simulink model "Filtering_PI_PreliminarySimulation"  (R2025a)
settings: Solver=VariableStepAuto  StartTime=0.0  StopTime=0.5  MaxStep=1e-4  RelTol=1e-3
undefined symbols (not defined in the file): D1, lagging, pulse
libraries: spsSeriesRLCBranchLib x43, spsGroundLib x17, spsMeanLib x1, spsMultimeterLib x1, slpidlib x1, spsPLL3phLib x1, spsPower3phInstantaneousLib x1, spsPulseGeneratorThyristor6PulseLib x1, spsRMSLib x1, simulink x1, spsThreePhaseProgrammableVoltageSourceLib x1, spsThreePhaseSeriesRLCBranchLib x1
settings Model: Creator=wz  LastModifiedBy=wz

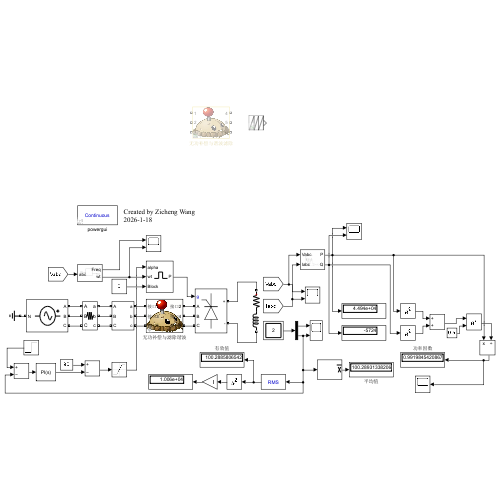
[thumbnail: Simulink's stored preview of the top-level diagram]
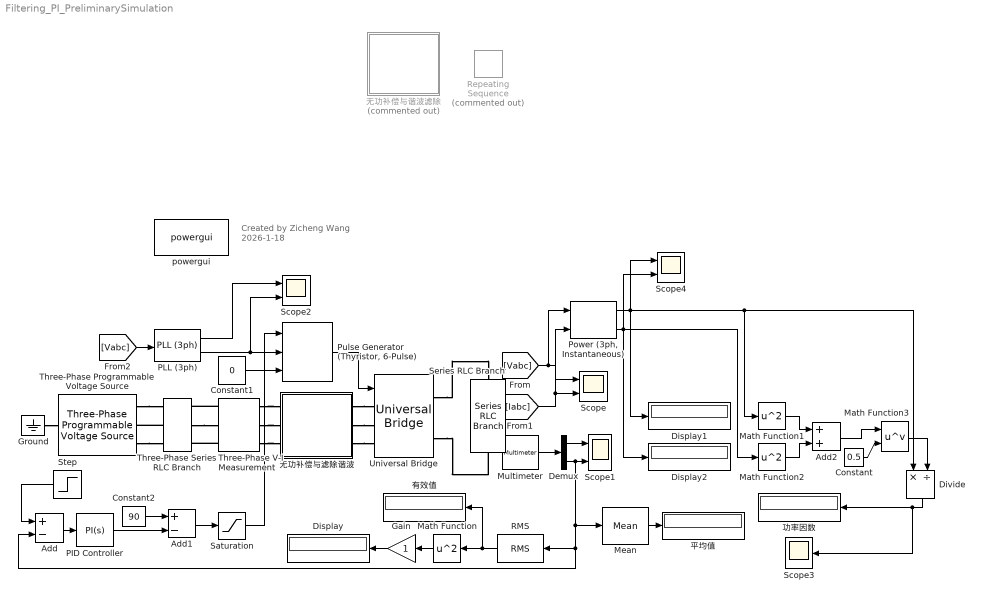
== system Filtering_PI_PreliminarySimulation ==
  note: Created by Zicheng Wang
      | 2026-1-18
  Add : Sum  Inputs=+-
  Add1 : Sum  Inputs=+-
  Add2 : Sum
  Constant : Constant  Value=0.5
  Constant1 : Constant  Value=0
  Constant2 : Constant  Value=90
  Demux : Demux  Outputs=2
  Display : Display
  Display1 : Display
  Display2 : Display
  Divide : Product  Inputs=*/
  Gain : Gain
  Ground : spsGroundLib/Ground  LConnTagsString=a
  Math Function : Math  Operator=square
  Math Function1 : Math  Operator=square
  Math Function2 : Math  Operator=square
  Math Function3 : Math  Operator=pow
  Mean : spsMeanLib/Mean  Freq=60  Vinit=0  Ts=0
  Multimeter : spsMultimeterLib/Multimeter  L=2  sel=[1 2]  yselected={}  Gain=[1 1]  OutputType=Complex  PlotAtSimulationStop=off  PhasorSimulation=off
  PID Controller : slpidlib/PID Controller  Controller=PI  Form=Parallel  TimeDomain=Continuous-time  UseExternalTs=off  SampleTime=-1  IntegratorMethod=Forward Euler  FilterMethod=Forward Euler  ControllerParametersSource=internal  P=2  I=0.5  UseKiTs=off  D=0  UseExternalDerivativeSource=off  N=100  UseFilter=on  TunerSelectOption=Transfer Function Based (PID Tuner App)  InitialConditionSource=internal  InitialConditionForIntegrator=0  InitialConditionForFilter=0  DifferentiatorICPrevScaledInput=0  ExternalReset=none  TrackingMode=off  Kt=1  LimitOutput=off  SatLimitsSource=internal  UpperSaturationLimit=inf  LowerSaturationLimit=-inf  LinearizeAsGain=on  AntiWindupMode=none  Kb=1  LimitIntegrator=off  UpperIntegratorSaturationLimit=inf  LowerIntegratorSaturationLimit=-inf  POutMin=[]  POutMax=[]  IOutMin=[]  IOutMax=[]  DOutMin=[]  DOutMax=[]  NOutMin=[]  NOutMax=[]  SumOutMin=[]  SumOutMax=[]  SaturationOutMin=[]  SaturationOutMax=[]  PParamMin=[]  PParamMax=[]  IParamMin=[]  IParamMax=[]  DParamMin=[]  DParamMax=[]  NParamMin=[]  NParamMax=[]  KbParamMin=[]  KbParamMax=[]  KtParamMin=[]  KtParamMax=[]  KbOutMin=[]  KbOutMax=[]  KtOutMin=[]  KtOutMax=[]  IntegratorOutMin=[]  IntegratorOutMax=[]  FilterOutMin=[]  FilterOutMax=[]  SumI1OutMin=[]  SumI1OutMax=[]  SumI2OutMin=[]  SumI2OutMax=[]  SumI3OutMin=[]  SumI3OutMax=[]  SumI4OutMin=[]  SumI4OutMax=[]  SumDOutMin=[]  SumDOutMax=[]  DifferentiatorOutMin=[]  DifferentiatorOutMax=[]  FilterDiffOutCoefMin=[]  FilterDiffOutCoefMax=[]  ReciprocalOutMin=[]  ReciprocalOutMax=[]  SumDenOutMin=[]  SumDenOutMax=[]  SumNumOutMin=[]  SumNumOutMax=[]  DivideOutMin=[]  DivideOutMax=[]  UdiffTsProdOutMin=[]  UdiffTsProdOutMax=[]  NTsProdOutMin=[]  NTsProdOutMax=[]  UintegralTsProdOutMin=[]  UintegralTsProdOutMax=[]  UngainTsProdOutMin=[]  UngainTsProdOutMax=[]  ClampingZeroOutDataTypeStr=Inherit: Inherit via back propagation  ClampingZeroOutMin=[]  ClampingZeroOutMax=[]  FilterDenConstantOutDataTypeStr=Inherit: Inherit via back propagation  FilterDenConstantOutMin=[]  FilterDenConstantOutMax=[]  PCopyOutDataTypeStr=Inherit: Inherit via back propagation  PCopyOutMin=[]  PCopyOutMax=[]  NCopyOutDataTypeStr=Inherit: Inherit via back propagation  NCopyOutMin=[]  NCopyOutMax=[]  IntegratorContinuousStateAttributes=''  IntegratorStateMustResolveToSignalObject=off  IntegratorRTWStateStorageClass=Auto  FilterContinuousStateAttributes=''  FilterStateMustResolveToSignalObject=off  FilterRTWStateStorageClass=Auto  ParallelPVariant=InternalParameters  IdealPVariant=Disabled  IVariant=InternalParameters  DVariant=Disabled  IntegratorVariant=Continuous  SatVariant=Disabled  AWVariant=Passthrough  PCopyVariant=Disabled  TRVariant=Disabled  FdbkBlocksVariant=Forward  IdealPFdbkVariant=Disabled  SatFdbkVariant=Disabled  DerivativeFilterVariant=Disabled  NVariant=Disabled  NCopyVariant=Disabled_SignalSpec  FilterICVariant=Disabled  IntegratorICVariant=InternalICs  ExternalResetVariant=Disabled  TRSumVariant=Passthrough  SumFdbkVariant=Disabled  SumVariant=Sum_PI  TsampFilterVariant=InternalTs  TsampNgainVariant=Passthrough  TsampIntegralVariant=Disabled_SignalSpec  ExternalSaturationOutDataTypeStr=Inherit: Same as second input  DerivativeSourceVariant=Disabled  PreIntVariant=InternalPreInt
  PLL (3ph) : spsPLL3phLib/PLL (3ph)  Fmin=49  Par_Init=[0, 50]  ParK=[180, 3200, 1]  TcD=1e-4  MaxRateChangeFreq=12  FilterCutOffFreq=25  Ts=0  AGC=on
  "Power (3ph, Instantaneous)" : spsPower3phInstantaneousLib/Power (3ph, Instantaneous)
  "Pulse Generator (Thyristor, 6-Pulse)" : spsPulseGeneratorThyristor6PulseLib/Pulse Generator (Thyristor, 6-Pulse)  GenType=6-pulse  Delta=D1 (lagging)  pwidth=60  Double_Pulse=off  Ts=0
      settings: LibrarySourceBlock=|
      | sps_lib/Power Electronics/Power Electronics Control/Pulse Generator
      | (Thyristor, 6-Pulse)
  RMS : spsRMSLib/RMS  TrueRMS=on  Freq=50  RMSInit=120  Ts=0
  Repeating Sequence : simulink/Sources/Repeating Sequence  Commented=on  rep_seq_t=[0 1/50]  rep_seq_y=[0 2*pi]
  Saturation : Saturate  UpperLimit=90  LowerLimit=0
  Scope{,1..2,4} (4 alike) : Scope  NumInputPorts=2
      Scope settings: ActiveDisplayYMinimum=-1  ActiveDisplayYMaximum=1
      Scope1 settings: ActiveDisplayYMinimum=-51.707918022923707  ActiveDisplayYMaximum=59.934540956922731
      Scope2 settings: ActiveDisplayYMinimum=-1  ActiveDisplayYMaximum=1  DataLoggingVariableName=ScopeData2
      Scope4 settings: ActiveDisplayYMinimum=-1  ActiveDisplayYMaximum=1  DataLoggingVariableName=ScopeData4
  Scope3 : Scope
      settings: ActiveDisplayYMinimum=0.98403716767059757  ActiveDisplayYMaximum=0.9967412923994573  DataLoggingVariableName=ScopeData3
  Series RLC Branch : spsSeriesRLCBranchLib/Series RLC Branch  LConnTagsString=__new0  RConnTagsString=__new0  BranchType=RL  Resistance=0.01  Inductance=0.025  SetiL0=off  InitialCurrent=0  Capacitance=1e-6  Setx0=off  InitialVoltage=0  Measurements=Branch voltage and current
  Step : Step  Time=0.02  After=105  SampleTime=0
  Three-Phase Programmable Voltage Source : spsThreePhaseProgrammableVoltageSourceLib/Three-Phase Programmable Voltage Source  PositiveSequence="[380  0 50]"  VariationEntity=None  VariationType=Table of time-amplitude pairs  VariationTypeAlt=Step  VariationStep=0.5  VariationRate=10  VariationMagnitude=0.3  VariationFrequency=2  VariationTiming=[1 2]  VariationPhaseA=off  Amplitudes=[1 0.8 1.2 1.0]  TimeValues=[0 0.1 0.15 0.2]  HarmonicGeneration=off  HarmonicA=[3 0.2 -25 0]  HarmonicB=[2 0.15 35 2]  Timing="[0.05  3]"  BusType=swing  Pref=0  Qref=0  Qmin=-inf  Qmax=inf
  Three-Phase Series RLC Branch : spsThreePhaseSeriesRLCBranchLib/Three-Phase Series RLC Branch  LConnTagsString=A|B|C  RConnTagsString=A|B|C  BranchType=R  Resistance=0.01  Inductance=1e-3  Capacitance=1e-6  Measurements=None
  Three-Phase V-I Measurement : spsThreePhaseVIMeasurementLib/Three-Phase V-I Measurement  VoltageMeasurement=phase-to-ground  SetLabelV=on  LabelV=Vabc  Vpu=off  VpuLL=off  CurrentMeasurement=yes  SetLabelI=on  LabelI=Iabc  Ipu=off  Pbase=100e6  Vbase=500e3  OutputType=Complex  PhasorSimulation=off  PSBequivalent=0
  Universal Bridge : spsUniversalBridgeLib/Universal Bridge  Arms=3  SnubberResistance=1e5  SnubberCapacitance=inf  Device=Thyristors  Ron=1e-3  Lon=0  ForwardVoltages="[  0  0  ]"  ForwardVoltage=0  GTOparameters=[ 10e-6 , 20e-6 ]  IGBTparameters=[ 1e-6 , 2e-6 ]  Measurements=None  Measurements_2=None  converterType=Rectifier
  powergui : sps_lib/powergui  Priority=1  SimulationMode=Continuous  SampleTime=50e-6  frequency=60  Iterations=50  frequencyindice=50  Pbase=100e6  ErrMax=1e-4  UnitsV=kV  UnitsW=MW  buscounter=0  FunctionMessages=off  echomessages=off  EnableUseOfTLC=off  CurrentSourceSwitches=off  DisableSnubberDevices=off  DisableRonSwitches=off  DisableVfSwitches=off  DisplayEquations=off  AutomaticDiscreteSolvers=off  SolverType=Tustin/Backward Euler (TBE)  Interpol=off  ExternalGateDelay=off  methode=off  Ts=100  x0status=blocks  SPID=on  SwTol=0  HookPort=off  NonlinearTolerance=1e-4  nMaxIteration=100  ContinueOnMaxIteration=off  RestoreLinks=warning  ResistiveCurrentMeasurement=off  Frange=[0:2:500]  Ylog=off  Xlog=on  ShowGrid=off  save=off  variable=ZData  structure=0  ZoomFFT=off  StartTime=0.0  cycles=1  DisplayStyle=1  fundamental=60  FreqAxis=off  MaxFrequency=1000  frequencyindicesteady=1  RmsSteady=1  display=off
  功率因数 : Display
  平均值 : Display
  无功补偿与滤除谐波 : Subsystem  mask{R0=1.2, R1=0.65, R2=0.65, R3=0.45, CLBQ1=1e-2, RLBQ1=0.0001, LLBQ1=4.05284734569351, CLBQ2=3e-4, RLBQ2=1e-6, LLBQ2=0.000689259752668965, CLBQ3=3e-3, RLBQ3=1e-4, LLBQ3=0.000279121718022969, CLBQ4=5e-3, RLBQ4=0.3, LLBQ4=0.0059953363101975/5, CLBQ5=10, RLBQ5=50, LLBQ5=3.50592330942345}
      mask prompts: R0 "R0value1"; R1 "R0value2"; R2 "R0value3"; R3 "R0value4"; CLBQ1 "CLBQvalue1"; RLBQ1 "RLBQvalue1"; LLBQ1 "LLBQvalue1"; CLBQ2 "CLBQvalue2"; RLBQ2 "RLBQvalue2"; LLBQ2 "LLBQvalue2"; CLBQ3 "CLBQvalue3"; RLBQ3 "RLBQvalue3"; LLBQ3 "LLBQvalue3"; CLBQ4 "CLBQvalue4"; RLBQ4 "RLBQvalue4"; LLBQ4 "LLBQvalue4"; CLBQ5 "CLBQvalue5"; RLBQ5 "RLBQvalue5"; LLBQ5 "LLBQvalue5"
      mask Display: image('微信图片_20240530165846.jpg');
  无功补偿与谐波滤除 : Subsystem  Commented=on
      mask DialogControl DescTextVar Prompt: 单调
      mask DialogControl ParameterGroupVar Prompt: 参数
      mask Display: image('微信图片_20240530165846.jpg');
  有效值 : Display
  wires:
  Constant1/1 -> "Pulse Generator (Thyristor, 6-Pulse)"/3
  [Vabc] -> "Power (3ph, Instantaneous)"/1, Scope/1
  [Iabc] -> "Power (3ph, Instantaneous)"/2, Scope/2
  PLL (3ph)/2 -> Scope2/2, "Pulse Generator (Thyristor, 6-Pulse)"/2
  "Pulse Generator (Thyristor, 6-Pulse)"/1 -> Universal Bridge/1
  [Vabc] -> PLL (3ph)/1
  PLL (3ph)/1 -> Scope2/1
  Multimeter/1 -> Demux/1
  Demux/1 -> Scope1/1
  Demux/2 -> Mean/1, Add/2, RMS/1, Scope1/2
  Add/1 -> PID Controller/1
  PID Controller/1 -> Add1/2
  Constant2/1 -> Add1/1
  Add1/1 -> Saturation/1
  Saturation/1 -> "Pulse Generator (Thyristor, 6-Pulse)"/1
  RMS/1 -> 有效值/1, Math Function/1
  Math Function/1 -> Gain/1
  Gain/1 -> Display/1
  "Power (3ph, Instantaneous)"/1 -> Scope4/1, Divide/1, Math Function1/1, Display1/1
  "Power (3ph, Instantaneous)"/2 -> Scope4/2, Math Function2/1, Display2/1
  Step/1 -> Add/1
  Math Function1/1 -> Add2/1
  Math Function2/1 -> Add2/2
  Add2/1 -> Math Function3/1
  Constant/1 -> Math Function3/2
  Math Function3/1 -> Divide/2
  Divide/1 -> Scope3/1, 功率因数/1
  Mean/1 -> 平均值/1
  connections:
  Universal Bridge/RConn1 -- Series RLC Branch/LConn1
  Universal Bridge/RConn2 -- Series RLC Branch/RConn1
  Ground/LConn1 -- Three-Phase Programmable Voltage Source/LConn1
  无功补偿与滤除谐波/RConn1 -- Universal Bridge/LConn1
  无功补偿与滤除谐波/RConn2 -- Universal Bridge/LConn2
  无功补偿与滤除谐波/RConn3 -- Universal Bridge/LConn3
  Three-Phase V-I Measurement/RConn1 -- 无功补偿与滤除谐波/LConn1
  Three-Phase V-I Measurement/RConn2 -- 无功补偿与滤除谐波/LConn2
  Three-Phase V-I Measurement/RConn3 -- 无功补偿与滤除谐波/LConn3
  Three-Phase Programmable Voltage Source/RConn1 -- Three-Phase Series RLC Branch/LConn1
  Three-Phase V-I Measurement/LConn1 -- Three-Phase Series RLC Branch/RConn1
  Three-Phase Series RLC Branch/LConn2 -- Three-Phase Programmable Voltage Source/RConn2
  Three-Phase Programmable Voltage Source/RConn3 -- Three-Phase Series RLC Branch/LConn3
  Three-Phase Series RLC Branch/RConn2 -- Three-Phase V-I Measurement/LConn2
  Three-Phase V-I Measurement/LConn3 -- Three-Phase Series RLC Branch/RConn3

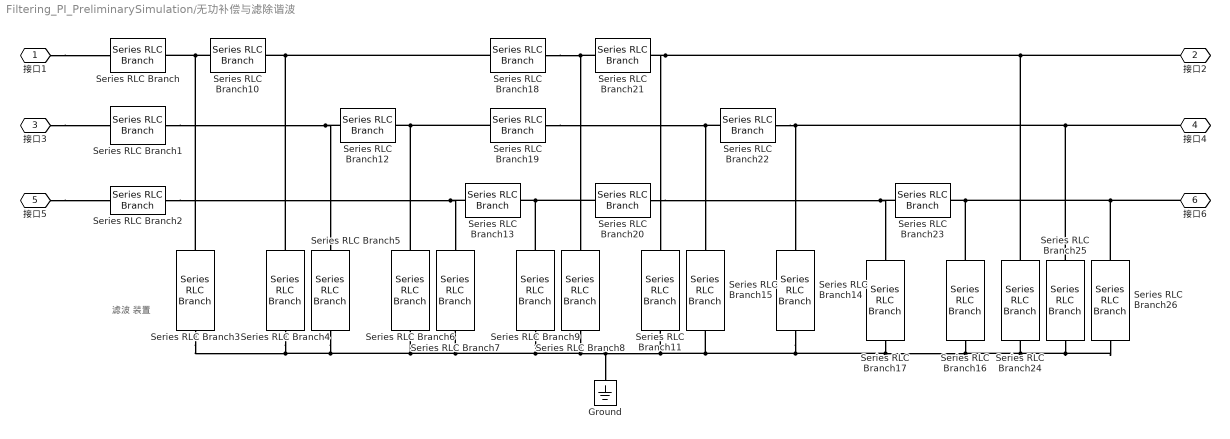
== system Filtering_PI_PreliminarySimulation/无功补偿与滤除谐波 ==
  note: 滤波
      | 装置
  Ground : spsGroundLib/Ground  LConnTagsString=a
  Series RLC Branch : spsSeriesRLCBranchLib/Series RLC Branch  LConnTagsString=__new0  RConnTagsString=__new0  BranchType=R  Resistance=R0  Inductance=1e-3  SetiL0=off  InitialCurrent=0  Capacitance=1e-6  Setx0=off  InitialVoltage=0  Measurements=None
  Series RLC Branch1 : spsSeriesRLCBranchLib/Series RLC Branch  LConnTagsString=__new0  RConnTagsString=__new0  BranchType=R  Resistance=R0  Inductance=1e-3  SetiL0=off  InitialCurrent=0  Capacitance=1e-6  Setx0=off  InitialVoltage=0  Measurements=None
  Series RLC Branch10 : spsSeriesRLCBranchLib/Series RLC Branch  LConnTagsString=__new0  RConnTagsString=__new0  BranchType=R  Resistance=R1  Inductance=1e-3  SetiL0=off  InitialCurrent=0  Capacitance=1e-6  Setx0=off  InitialVoltage=0  Measurements=None
  Series RLC Branch11 : spsSeriesRLCBranchLib/Series RLC Branch  LConnTagsString=__new0  RConnTagsString=__new0  BranchType=RLC  Resistance=RLBQ4  Inductance=LLBQ4  SetiL0=off  InitialCurrent=0  Capacitance=CLBQ4  Setx0=off  InitialVoltage=0  Measurements=None
  Series RLC Branch12 : spsSeriesRLCBranchLib/Series RLC Branch  LConnTagsString=__new0  RConnTagsString=__new0  BranchType=R  Resistance=R1  Inductance=1e-3  SetiL0=off  InitialCurrent=0  Capacitance=1e-6  Setx0=off  InitialVoltage=0  Measurements=None
  Series RLC Branch13 : spsSeriesRLCBranchLib/Series RLC Branch  LConnTagsString=__new0  RConnTagsString=__new0  BranchType=R  Resistance=R1  Inductance=1e-3  SetiL0=off  InitialCurrent=0  Capacitance=1e-6  Setx0=off  InitialVoltage=0  Measurements=None
  Series RLC Branch14 : spsSeriesRLCBranchLib/Series RLC Branch  LConnTagsString=__new0  RConnTagsString=__new0  BranchType=RLC  Resistance=RLBQ4  Inductance=LLBQ4  SetiL0=off  InitialCurrent=0  Capacitance=CLBQ4  Setx0=off  InitialVoltage=0  Measurements=None
  Series RLC Branch15 : spsSeriesRLCBranchLib/Series RLC Branch  LConnTagsString=__new0  RConnTagsString=__new0  BranchType=RLC  Resistance=RLBQ3  Inductance=LLBQ3  SetiL0=off  InitialCurrent=0  Capacitance=CLBQ3  Setx0=off  InitialVoltage=0  Measurements=None
  Series RLC Branch16 : spsSeriesRLCBranchLib/Series RLC Branch  LConnTagsString=__new0  RConnTagsString=__new0  BranchType=RLC  Resistance=RLBQ4  Inductance=LLBQ4  SetiL0=off  InitialCurrent=0  Capacitance=CLBQ4  Setx0=off  InitialVoltage=0  Measurements=None
  Series RLC Branch17 : spsSeriesRLCBranchLib/Series RLC Branch  LConnTagsString=__new0  RConnTagsString=__new0  BranchType=RLC  Resistance=RLBQ3  Inductance=LLBQ3  SetiL0=off  InitialCurrent=0  Capacitance=CLBQ3  Setx0=off  InitialVoltage=0  Measurements=None
  Series RLC Branch18 : spsSeriesRLCBranchLib/Series RLC Branch  LConnTagsString=__new0  RConnTagsString=__new0  BranchType=R  Resistance=R2  Inductance=1e-3  SetiL0=off  InitialCurrent=0  Capacitance=1e-6  Setx0=off  InitialVoltage=0  Measurements=None
  Series RLC Branch19 : spsSeriesRLCBranchLib/Series RLC Branch  LConnTagsString=__new0  RConnTagsString=__new0  BranchType=R  Resistance=R2  Inductance=1e-3  SetiL0=off  InitialCurrent=0  Capacitance=1e-6  Setx0=off  InitialVoltage=0  Measurements=None
  Series RLC Branch2 : spsSeriesRLCBranchLib/Series RLC Branch  LConnTagsString=__new0  RConnTagsString=__new0  BranchType=R  Resistance=R0  Inductance=1e-3  SetiL0=off  InitialCurrent=0  Capacitance=1e-6  Setx0=off  InitialVoltage=0  Measurements=None
  Series RLC Branch20 : spsSeriesRLCBranchLib/Series RLC Branch  LConnTagsString=__new0  RConnTagsString=__new0  BranchType=R  Resistance=R2  Inductance=1e-3  SetiL0=off  InitialCurrent=0  Capacitance=1e-6  Setx0=off  InitialVoltage=0  Measurements=None
  Series RLC Branch21 : spsSeriesRLCBranchLib/Series RLC Branch  LConnTagsString=__new0  RConnTagsString=__new0  BranchType=R  Resistance=R3  Inductance=1e-3  SetiL0=off  InitialCurrent=0  Capacitance=1e-6  Setx0=off  InitialVoltage=0  Measurements=None
  Series RLC Branch22 : spsSeriesRLCBranchLib/Series RLC Branch  LConnTagsString=__new0  RConnTagsString=__new0  BranchType=R  Resistance=R3  Inductance=1e-3  SetiL0=off  InitialCurrent=0  Capacitance=1e-6  Setx0=off  InitialVoltage=0  Measurements=None
  Series RLC Branch23 : spsSeriesRLCBranchLib/Series RLC Branch  LConnTagsString=__new0  RConnTagsString=__new0  BranchType=R  Resistance=R3  Inductance=1e-3  SetiL0=off  InitialCurrent=0  Capacitance=1e-6  Setx0=off  InitialVoltage=0  Measurements=None
  Series RLC Branch24 : spsSeriesRLCBranchLib/Series RLC Branch  LConnTagsString=__new0  RConnTagsString=__new0  BranchType=RLC  Resistance=RLBQ5  Inductance=LLBQ5  SetiL0=off  InitialCurrent=0  Capacitance=CLBQ5  Setx0=off  InitialVoltage=0  Measurements=None
  Series RLC Branch25 : spsSeriesRLCBranchLib/Series RLC Branch  LConnTagsString=__new0  RConnTagsString=__new0  BranchType=RLC  Resistance=RLBQ5  Inductance=LLBQ5  SetiL0=off  InitialCurrent=0  Capacitance=CLBQ5  Setx0=off  InitialVoltage=0  Measurements=None
  Series RLC Branch26 : spsSeriesRLCBranchLib/Series RLC Branch  LConnTagsString=__new0  RConnTagsString=__new0  BranchType=RLC  Resistance=RLBQ5  Inductance=LLBQ5  SetiL0=off  InitialCurrent=0  Capacitance=CLBQ5  Setx0=off  InitialVoltage=0  Measurements=None
  Series RLC Branch3 : spsSeriesRLCBranchLib/Series RLC Branch  LConnTagsString=__new0  RConnTagsString=__new0  BranchType=RLC  Resistance=RLBQ1  Inductance=LLBQ1  SetiL0=off  InitialCurrent=0  Capacitance=CLBQ1  Setx0=off  InitialVoltage=0  Measurements=None
  Series RLC Branch4 : spsSeriesRLCBranchLib/Series RLC Branch  LConnTagsString=__new0  RConnTagsString=__new0  BranchType=RLC  Resistance=RLBQ2  Inductance=LLBQ2  SetiL0=off  InitialCurrent=0  Capacitance=CLBQ2  Setx0=off  InitialVoltage=0  Measurements=None
  Series RLC Branch5 : spsSeriesRLCBranchLib/Series RLC Branch  LConnTagsString=__new0  RConnTagsString=__new0  BranchType=RLC  Resistance=RLBQ1  Inductance=LLBQ1  SetiL0=off  InitialCurrent=0  Capacitance=CLBQ1  Setx0=off  InitialVoltage=0  Measurements=None
  Series RLC Branch6 : spsSeriesRLCBranchLib/Series RLC Branch  LConnTagsString=__new0  RConnTagsString=__new0  BranchType=RLC  Resistance=RLBQ2  Inductance=LLBQ2  SetiL0=off  InitialCurrent=0  Capacitance=CLBQ2  Setx0=off  InitialVoltage=0  Measurements=None
  Series RLC Branch7 : spsSeriesRLCBranchLib/Series RLC Branch  LConnTagsString=__new0  RConnTagsString=__new0  BranchType=RLC  Resistance=RLBQ1  Inductance=LLBQ1  SetiL0=off  InitialCurrent=0  Capacitance=CLBQ1  Setx0=off  InitialVoltage=0  Measurements=None
  Series RLC Branch8 : spsSeriesRLCBranchLib/Series RLC Branch  LConnTagsString=__new0  RConnTagsString=__new0  BranchType=RLC  Resistance=RLBQ3  Inductance=LLBQ3  SetiL0=off  InitialCurrent=0  Capacitance=CLBQ3  Setx0=off  InitialVoltage=0  Measurements=None
  Series RLC Branch9 : spsSeriesRLCBranchLib/Series RLC Branch  LConnTagsString=__new0  RConnTagsString=__new0  BranchType=RLC  Resistance=RLBQ2  Inductance=LLBQ2  SetiL0=off  InitialCurrent=0  Capacitance=CLBQ2  Setx0=off  InitialVoltage=0  Measurements=None
  接口1 : PMIOPort  Side=Left
  接口2 : PMIOPort  Port=2  Side=Right
  接口3 : PMIOPort  Port=3  Side=Left
  接口4 : PMIOPort  Port=4  Side=Right
  接口5 : PMIOPort  Port=5  Side=Left
  接口6 : PMIOPort  Port=6  Side=Right
  connections:
  Series RLC Branch3/LConn1 -- Series RLC Branch10/LConn1 -- Series RLC Branch/RConn1
  Series RLC Branch1/RConn1 -- Series RLC Branch12/LConn1 -- Series RLC Branch5/LConn1
  Series RLC Branch2/RConn1 -- Series RLC Branch13/LConn1 -- Series RLC Branch7/LConn1
  接口1/RConn1 -- Series RLC Branch/LConn1
  接口3/RConn1 -- Series RLC Branch1/LConn1
  接口5/RConn1 -- Series RLC Branch2/LConn1
  Series RLC Branch25/RConn1 -- Series RLC Branch26/RConn1 -- Series RLC Branch24/RConn1 -- Series RLC Branch16/RConn1 -- Series RLC Branch17/RConn1 -- Series RLC Branch15/RConn1 -- Series RLC Branch3/RConn1 -- Series RLC Branch4/RConn1 -- Series RLC Branch5/RConn1 -- Series RLC Branch6/RConn1 -- Series RLC Branch7/RConn1 -- Series RLC Branch9/RConn1 -- Series RLC Branch8/RConn1 -- Ground/LConn1 -- Series RLC Branch11/RConn1 -- Series RLC Branch14/RConn1
  Series RLC Branch18/RConn1 -- Series RLC Branch21/LConn1 -- Series RLC Branch8/LConn1
  Series RLC Branch6/LConn1 -- Series RLC Branch19/LConn1 -- Series RLC Branch12/RConn1
  Series RLC Branch20/RConn1 -- Series RLC Branch23/LConn1 -- Series RLC Branch17/LConn1
  Series RLC Branch4/LConn1 -- Series RLC Branch18/LConn1 -- Series RLC Branch10/RConn1
  Series RLC Branch19/RConn1 -- Series RLC Branch22/LConn1 -- Series RLC Branch15/LConn1
  Series RLC Branch9/LConn1 -- Series RLC Branch20/LConn1 -- Series RLC Branch13/RConn1
  Series RLC Branch21/RConn1 -- Series RLC Branch24/LConn1 -- 接口2/RConn1 -- Series RLC Branch11/LConn1
  Series RLC Branch22/RConn1 -- Series RLC Branch25/LConn1 -- 接口4/RConn1 -- Series RLC Branch14/LConn1
  Series RLC Branch16/LConn1 -- Series RLC Branch26/LConn1 -- 接口6/RConn1 -- Series RLC Branch23/RConn1

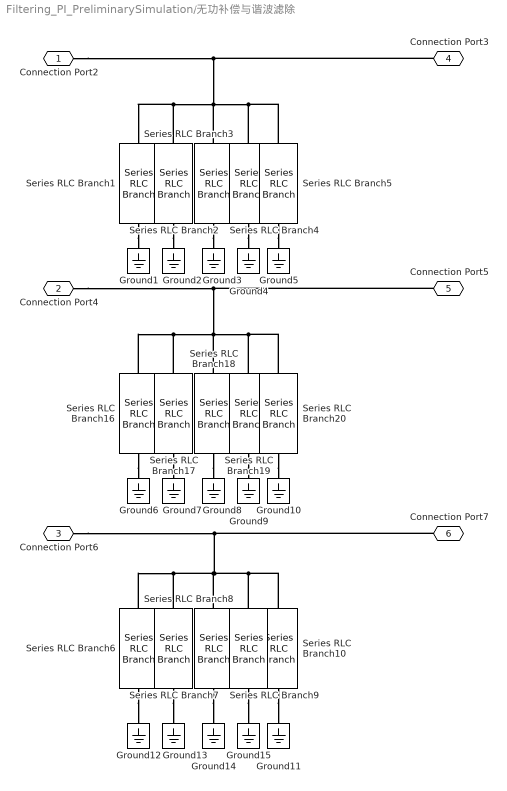
== system Filtering_PI_PreliminarySimulation/无功补偿与谐波滤除 ==
  Ground{1..15} (15 alike) : spsGroundLib/Ground  LConnTagsString=a
  Series RLC Branch1 : spsSeriesRLCBranchLib/Series RLC Branch  LConnTagsString=__new0  RConnTagsString=__new0  BranchType=RLC  Resistance=0.0001  Inductance=4.05285  SetiL0=off  InitialCurrent=0  Capacitance=0.01  Setx0=off  InitialVoltage=0  Measurements=None
  Series RLC Branch10 : spsSeriesRLCBranchLib/Series RLC Branch  LConnTagsString=__new0  RConnTagsString=__new0  BranchType=RLC  Resistance=1  Inductance=3.50592  SetiL0=off  InitialCurrent=0  Capacitance=5  Setx0=off  InitialVoltage=0  Measurements=None
  Series RLC Branch16 : spsSeriesRLCBranchLib/Series RLC Branch  LConnTagsString=__new0  RConnTagsString=__new0  BranchType=RLC  Resistance=0.0001  Inductance=4.05285  SetiL0=off  InitialCurrent=0  Capacitance=0.01  Setx0=off  InitialVoltage=0  Measurements=None
  Series RLC Branch17 : spsSeriesRLCBranchLib/Series RLC Branch  LConnTagsString=__new0  RConnTagsString=__new0  BranchType=RLC  Resistance=0.00001  Inductance=0.00069  SetiL0=off  InitialCurrent=0  Capacitance=0.0003  Setx0=off  InitialVoltage=0  Measurements=None
  Series RLC Branch18 : spsSeriesRLCBranchLib/Series RLC Branch  LConnTagsString=__new0  RConnTagsString=__new0  BranchType=RLC  Resistance=0.0001  Inductance=0.00028  SetiL0=off  InitialCurrent=0  Capacitance=0.003  Setx0=off  InitialVoltage=0  Measurements=None
  Series RLC Branch19 : spsSeriesRLCBranchLib/Series RLC Branch  LConnTagsString=__new0  RConnTagsString=__new0  BranchType=RLC  Resistance=0.3  Inductance=0.006  SetiL0=off  InitialCurrent=0  Capacitance=0.005  Setx0=off  InitialVoltage=0  Measurements=None
  Series RLC Branch2 : spsSeriesRLCBranchLib/Series RLC Branch  LConnTagsString=__new0  RConnTagsString=__new0  BranchType=RLC  Resistance=0.00001  Inductance=0.00069  SetiL0=off  InitialCurrent=0  Capacitance=0.0003  Setx0=off  InitialVoltage=0  Measurements=None
  Series RLC Branch20 : spsSeriesRLCBranchLib/Series RLC Branch  LConnTagsString=__new0  RConnTagsString=__new0  BranchType=RLC  Resistance=1  Inductance=3.50592  SetiL0=off  InitialCurrent=0  Capacitance=5  Setx0=off  InitialVoltage=0  Measurements=None
  Series RLC Branch3 : spsSeriesRLCBranchLib/Series RLC Branch  LConnTagsString=__new0  RConnTagsString=__new0  BranchType=RLC  Resistance=0.0001  Inductance=0.00028  SetiL0=off  InitialCurrent=0  Capacitance=0.003  Setx0=off  InitialVoltage=0  Measurements=None
  Series RLC Branch4 : spsSeriesRLCBranchLib/Series RLC Branch  LConnTagsString=__new0  RConnTagsString=__new0  BranchType=RLC  Resistance=0.3  Inductance=0.006  SetiL0=off  InitialCurrent=0  Capacitance=0.005  Setx0=off  InitialVoltage=0  Measurements=None
  Series RLC Branch5 : spsSeriesRLCBranchLib/Series RLC Branch  LConnTagsString=__new0  RConnTagsString=__new0  BranchType=RLC  Resistance=1  Inductance=3.50592  SetiL0=off  InitialCurrent=0  Capacitance=5  Setx0=off  InitialVoltage=0  Measurements=None
  Series RLC Branch6 : spsSeriesRLCBranchLib/Series RLC Branch  LConnTagsString=__new0  RConnTagsString=__new0  BranchType=RLC  Resistance=0.0001  Inductance=4.05285  SetiL0=off  InitialCurrent=0  Capacitance=0.01  Setx0=off  InitialVoltage=0  Measurements=None
  Series RLC Branch7 : spsSeriesRLCBranchLib/Series RLC Branch  LConnTagsString=__new0  RConnTagsString=__new0  BranchType=RLC  Resistance=0.00001  Inductance=0.00069  SetiL0=off  InitialCurrent=0  Capacitance=0.0003  Setx0=off  InitialVoltage=0  Measurements=None
  Series RLC Branch8 : spsSeriesRLCBranchLib/Series RLC Branch  LConnTagsString=__new0  RConnTagsString=__new0  BranchType=RLC  Resistance=0.0001  Inductance=0.00028  SetiL0=off  InitialCurrent=0  Capacitance=0.003  Setx0=off  InitialVoltage=0  Measurements=None
  Series RLC Branch9 : spsSeriesRLCBranchLib/Series RLC Branch  LConnTagsString=__new0  RConnTagsString=__new0  BranchType=RLC  Resistance=0.3  Inductance=0.006  SetiL0=off  InitialCurrent=0  Capacitance=0.005  Setx0=off  InitialVoltage=0  Measurements=None
  Connection Port2 : PMIOPort  Side=Left
  Connection Port4 : PMIOPort  Port=2  Side=Left
  Connection Port6 : PMIOPort  Port=3  Side=Left
  Connection Port3 : PMIOPort  Port=4  Side=Right
  Connection Port5 : PMIOPort  Port=5  Side=Right
  Connection Port7 : PMIOPort  Port=6  Side=Right
  connections:
  Connection Port7/RConn1 -- Connection Port6/RConn1 -- Series RLC Branch6/LConn1 -- Series RLC Branch7/LConn1 -- Series RLC Branch8/LConn1 -- Series RLC Branch10/LConn1 -- Series RLC Branch9/LConn1
  Series RLC Branch18/RConn1 -- Ground8/LConn1
  Connection Port4/RConn1 -- Connection Port5/RConn1 -- Series RLC Branch18/LConn1 -- Series RLC Branch17/LConn1 -- Series RLC Branch16/LConn1 -- Series RLC Branch20/LConn1 -- Series RLC Branch19/LConn1
  Series RLC Branch4/RConn1 -- Ground4/LConn1
  Series RLC Branch19/RConn1 -- Ground9/LConn1
  Series RLC Branch5/RConn1 -- Ground5/LConn1
  Series RLC Branch3/RConn1 -- Ground3/LConn1
  Series RLC Branch2/RConn1 -- Ground2/LConn1
  Series RLC Branch1/RConn1 -- Ground1/LConn1
  Series RLC Branch16/RConn1 -- Ground6/LConn1
  Series RLC Branch20/RConn1 -- Ground10/LConn1
  Series RLC Branch17/RConn1 -- Ground7/LConn1
  Series RLC Branch6/RConn1 -- Ground12/LConn1
  Series RLC Branch7/RConn1 -- Ground13/LConn1
  Series RLC Branch8/RConn1 -- Ground14/LConn1
  Series RLC Branch9/RConn1 -- Ground15/LConn1
  Series RLC Branch10/RConn1 -- Ground11/LConn1
  Series RLC Branch3/LConn1 -- Connection Port2/RConn1 -- Connection Port3/RConn1 -- Series RLC Branch2/LConn1 -- Series RLC Branch1/LConn1 -- Series RLC Branch5/LConn1 -- Series RLC Branch4/LConn1
